simulink model "Assignment_TestGen13"  (R2017b)
settings: Solver=FixedStepDiscrete  StartTime=0.0  StopTime=10.0  RelTol=1e-3
settings Model: Creator=hbourbou  LastModifiedBy=hbourbou
settings DebuggingCC: ParameterOverflowMsg=none

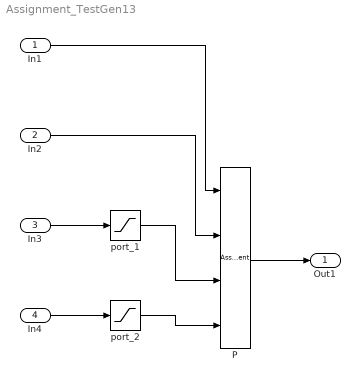
== system Assignment_TestGen13 ==
  In1 : Inport  OutDataTypeStr=single  PortDimensions=[3 3 3]
  In2 : Inport  Port=2  OutDataTypeStr=single  PortDimensions=[2 2 2]
  In3 : Inport  Port=3  OutMin=1  OutMax=2
  In4 : Inport  Port=4  OutMin=1  OutMax=2
  P : Assignment  NumberOfDimensions=3  DiagnosticForDimensions=Warning  IndexOptions=Index vector (port),Starting index (dialog),Starting index (port)  Indices=[],1,[]  OutputSizes=,,
  port_1 : Saturate  UpperLimit=2  LowerLimit=1
  port_2 : Saturate  UpperLimit=2  LowerLimit=1
  Out1 : Outport
  wires:
  In1/1 -> P/1
  In2/1 -> P/2
  port_1/1 -> P/3
  port_2/1 -> P/4
  In3/1 -> port_1/1
  In4/1 -> port_2/1
  P/1 -> Out1/1
